simulink model "x64_adc"  (R2016b)
settings: Solver=VariableStepAuto  StartTime=0.0  StopTime=10.0  RelTol=1e-3
libraries: xbsIndex_r4 x19
settings Model: Creator=qwerty40  LastModifiedBy=qwerty40

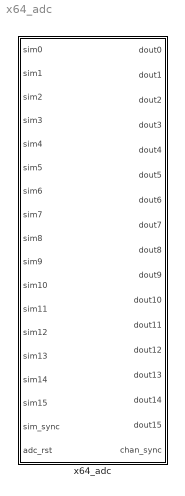
== system x64_adc ==
  x64_adc : Subsystem  Tag=xps:x64_adc  mask(x64_adc){adc_clk_rate=12, spi=off, ctrl_gpio=GPIO_A}
      mask prompts: adc_clk_rate "ADC clock rate (MHz)"; spi "Include SPI interface?"; ctrl_gpio "GPIO bank to use for control signals?"
      mask help: The ADC block converts analog inputs to digital outputs. Every clock cycle, the inputs are sampled and digitized to 8 bit binary point numbers in the range of [-1, 1) and are then output by the adc.
      mask init:
      | x64_adc_mask(gcb, 'spi', spi);
      mask Help: web([getenv('MLIB_DEVEL_PATH'), '/docs/_build/html/src/X64_adc.html'])
      mask TypeOptions ctrl_gpio: GPIO_A | GPIO_B

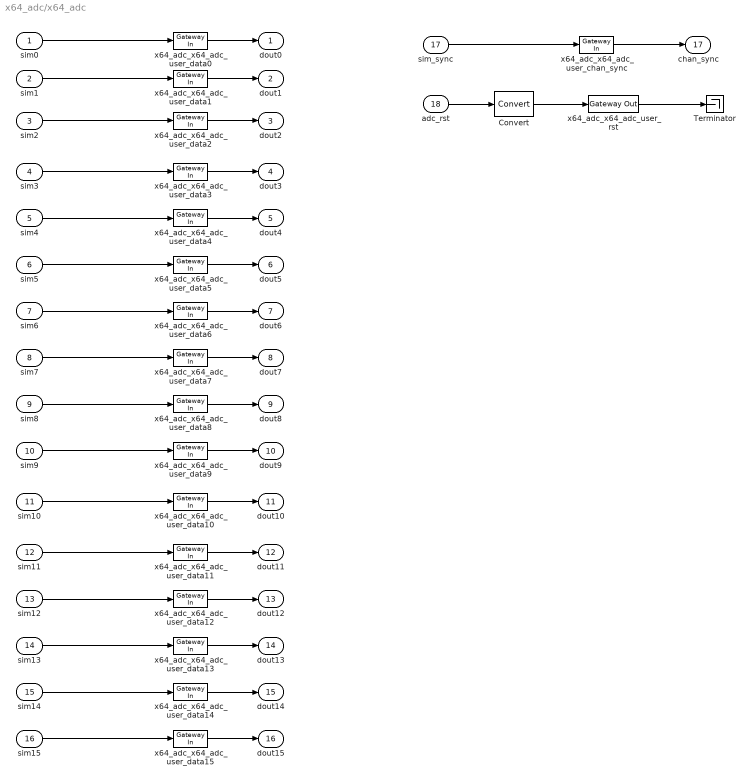
== system x64_adc/x64_adc ==
  sim0 : Inport
  sim1 : Inport  Port=2
  sim2 : Inport  Port=3
  sim3 : Inport  Port=4
  sim4 : Inport  Port=5
  sim5 : Inport  Port=6
  sim6 : Inport  Port=7
  sim7 : Inport  Port=8
  sim8 : Inport  Port=9
  sim9 : Inport  Port=10
  sim10 : Inport  Port=11
  sim11 : Inport  Port=12
  sim12 : Inport  Port=13
  sim13 : Inport  Port=14
  sim14 : Inport  Port=15
  sim15 : Inport  Port=16
  sim_sync : Inport  Port=17
  adc_rst : Inport  Port=18
  Convert : xbsIndex_r4/Convert  gui_display_data_type=Fixed-point  arith_type=Boolean  n_bits=16  bin_pt=14  float_type=Single  exp_bits=8  fraction_bits=24  quantization=Truncate  overflow=Wrap  en=off  latency=0  pipeline=off  dbl_ovrd=off  block_type=convert
      settings: block_version=11.4
  Terminator : Terminator
  x64_adc_x64_adc_user_chan_sync : xbsIndex_r4/Gateway In  gui_display_data_type=Fixed-point  arith_type=Unsigned  n_bits=8  bin_pt=0  preci_type=Single  exp_width=8  frac_width=24  rows=1  columns=1  quantization="Round  (unbiased: +/- Inf)"  overflow=Saturate  period=1  UseAsADC=off  ADCChannel='1'  interface=None  automatic_assignment=on  address_offset=hex2dec('00')  intf_name=''  intf_description=''  default_value=0  timing_constraint=None  locs_specified=off  LOCs={}  io_standard={}  inherit_from_input=off  hdl_port=on  dbl_ovrd=off  block_type=gatewayin
      settings: infoedit="Gateway in block.  Converts inputs of type Simulink integer, double and fixed point to  Xilinx fixed point type.<br><br>Hardware notes:  In hardware these blocks become top level input ports."  block_version=11.4
  x64_adc_x64_adc_user_data{0..15} (16 alike) : xbsIndex_r4/Gateway In  gui_display_data_type=Fixed-point  arith_type="Signed  (2's comp)"  n_bits=12  bin_pt=11  preci_type=Single  exp_width=8  frac_width=24  rows=1  columns=1  quantization="Round  (unbiased: +/- Inf)"  overflow=Saturate  period=1  UseAsADC=off  ADCChannel='1'  interface=None  automatic_assignment=on  address_offset=hex2dec('00')  intf_name=''  intf_description=''  default_value=0  timing_constraint=None  locs_specified=off  LOCs={}  io_standard={}  inherit_from_input=off  hdl_port=on  dbl_ovrd=off  block_type=gatewayin
      settings: infoedit="Gateway in block.  Converts inputs of type Simulink integer, double and fixed point to  Xilinx fixed point type.<br><br>Hardware notes:  In hardware these blocks become top level input ports."  block_version=11.4
  x64_adc_x64_adc_user_rst : xbsIndex_r4/Gateway Out  inherit_from_input=off  hdl_port=on  rows=1  columns=1  UseAsDAC=off  DACChannel='1'  interface=None  automatic_assignment=on  address_offset=hex2dec('00')  intf_name=''  intf_description=''  timing_constraint=None  locs_specified=off  LOCs={}  io_standard={}  block_type=gatewayout
      settings: infoedit="Gateway out block.  Converts Xilinx fixed point inputs into ouputs of type Simulink integer, double, or fixed point.<br><br>Hardware notes:  In hardware these blocks become top level output ports or are discarded, depending on how they are configured."  block_version=11.4
  dout0 : Outport
  dout1 : Outport  Port=2
  dout2 : Outport  Port=3
  dout3 : Outport  Port=4
  dout4 : Outport  Port=5
  dout5 : Outport  Port=6
  dout6 : Outport  Port=7
  dout7 : Outport  Port=8
  dout8 : Outport  Port=9
  dout9 : Outport  Port=10
  dout10 : Outport  Port=11
  dout11 : Outport  Port=12
  dout12 : Outport  Port=13
  dout13 : Outport  Port=14
  dout14 : Outport  Port=15
  dout15 : Outport  Port=16
  chan_sync : Outport  Port=17
  wires:
  x64_adc_x64_adc_user_data1/1 -> dout1/1
  sim1/1 -> x64_adc_x64_adc_user_data1/1
  Convert/1 -> x64_adc_x64_adc_user_rst/1
  x64_adc_x64_adc_user_rst/1 -> Terminator/1
  adc_rst/1 -> Convert/1
  x64_adc_x64_adc_user_chan_sync/1 -> chan_sync/1
  sim_sync/1 -> x64_adc_x64_adc_user_chan_sync/1
  x64_adc_x64_adc_user_data15/1 -> dout15/1
  sim15/1 -> x64_adc_x64_adc_user_data15/1
  x64_adc_x64_adc_user_data14/1 -> dout14/1
  sim14/1 -> x64_adc_x64_adc_user_data14/1
  x64_adc_x64_adc_user_data13/1 -> dout13/1
  sim13/1 -> x64_adc_x64_adc_user_data13/1
  x64_adc_x64_adc_user_data12/1 -> dout12/1
  sim12/1 -> x64_adc_x64_adc_user_data12/1
  x64_adc_x64_adc_user_data11/1 -> dout11/1
  sim11/1 -> x64_adc_x64_adc_user_data11/1
  x64_adc_x64_adc_user_data10/1 -> dout10/1
  sim10/1 -> x64_adc_x64_adc_user_data10/1
  x64_adc_x64_adc_user_data9/1 -> dout9/1
  sim9/1 -> x64_adc_x64_adc_user_data9/1
  x64_adc_x64_adc_user_data8/1 -> dout8/1
  sim8/1 -> x64_adc_x64_adc_user_data8/1
  x64_adc_x64_adc_user_data7/1 -> dout7/1
  sim7/1 -> x64_adc_x64_adc_user_data7/1
  x64_adc_x64_adc_user_data6/1 -> dout6/1
  sim6/1 -> x64_adc_x64_adc_user_data6/1
  x64_adc_x64_adc_user_data5/1 -> dout5/1
  sim5/1 -> x64_adc_x64_adc_user_data5/1
  x64_adc_x64_adc_user_data4/1 -> dout4/1
  sim4/1 -> x64_adc_x64_adc_user_data4/1
  x64_adc_x64_adc_user_data3/1 -> dout3/1
  sim3/1 -> x64_adc_x64_adc_user_data3/1
  x64_adc_x64_adc_user_data2/1 -> dout2/1
  sim2/1 -> x64_adc_x64_adc_user_data2/1
  x64_adc_x64_adc_user_data0/1 -> dout0/1
  sim0/1 -> x64_adc_x64_adc_user_data0/1
  ? -> ?
  ? -> ?
  ? -> ?
  ? -> ?
